simulink model "HLS_design"  (R2023a)
settings: Solver=VariableStepAuto  StartTime=0.0  StopTime=0  RelTol=1e-3  EnableMultiTasking=on
undefined symbols (not defined in the file): A, AXI4, N, Stream, xc7k325tffg900
libraries: hlsBasic x2, Sobeledge_lib x2, dspvision x1, vmcUtilities x1, hlsUtilities x1, visionsinks x1
settings Model: Creator=dvancamp  LastModifiedBy=robg
settings SolverCC: AlgebraicLoopSolver=TrustRegion
settings DataIOCC: LimitDataPoints=on  ReturnWorkspaceOutputs=off
settings OptimizationCC: LifeSpan=inf
settings DebuggingCC: UnconnectedInputMsg=warning  UnconnectedOutputMsg=warning  UnconnectedLineMsg=warning  AllowSymbolicDim=off  SFUnexpectedBacktrackingDiag=warning  SFNoUnconditionalDefaultTransitionDiag=warning  ArithmeticOperatorsInVariantConditions=warning
settings ModelReferenceCC: EnableRefExpFcnMdlSchedulingChecks=on  PropagateSignalLabelsOutOfModel=off
settings SFSimCC: SimUseLocalCustomCode=off  CustomCodeUndefinedFunction=UseInterfaceOnly
settings RTWCC: RTWUseLocalCustomCode=off
settings CodeAppCC: StateflowObjectComments=on
settings GRTTargetCC: TargetLangStandard=C89/C90 (ANSI)
settings ConfigComp: CovMetricSettings=dw  CovSaveCumulativeToWorkspaceVar=on  CovSaveSingleToWorkspaceVar=on  CovExternalEMLEnable=off

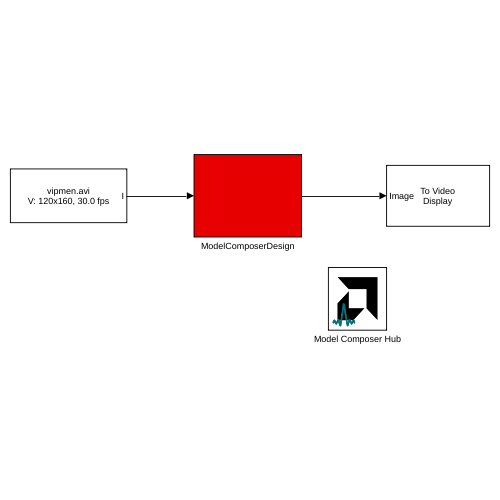
[thumbnail: Simulink's stored preview of the top-level diagram]
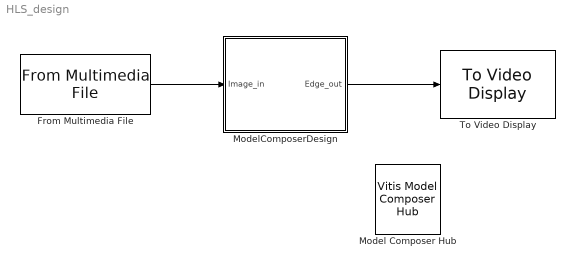
== system HLS_design ==
  From Multimedia File : dspvision/From Multimedia File  inputFilename=vipmen.avi  readRange=[1 Inf]  loop=on  numPlays=inf  outputStreams=Video only  videoDataType=uint8  audioDataType=double  inheritSampleTime=off  userDefinedSampleTime=1/30  noAudioOutput=off  isIntensityVideo=off  fourcc=Intensity  colorVideoFormat=One multidimensional signal  outputEOF=off  dataOrg=Column-major  audioFrameSize=1024  computeAudioFrameSize=off  outSamplingMode=Sample based
  Model Composer Hub : vmcUtilities/Vitis Model Composer Hub  Tag=genX  Description=Performs multiplication  CodeGeneration=off  SubsystemName=ModelComposerDesign  StartColumn=1  NumberOfColumns=1  TargetDirectory=code_HLS  exportDesign=off  analyzeDesign=off  validateDesignOnHw=off  ExportType=System Generator  IpVendor=xilinx.com  IpLibrary=hls  IpVersion=1.0  IpHWLanguage=Verilog  AieCompilerOptions={}  AieSimulatorOptions={}  CreateTestbench=off  TestbenchStackSize=10  RunRtlSim=off  RunCSim=off  RunAieSim=off  AieSimTimeout=50000  RunAieSimProfiling=off  LaunchVitisAnalyzer=off  PlotOutput=off  RunX86Sim=on  X86SimTimeout=10  GenHwImage=off  GenLibadfXo=off  GenHwValidationCode=off  PlatformType=Not Specified  HwSystemType=Baremetal  HwValidationTarget=hw  ProjDevice=Kintex-7 KC705 Evaluation Platform (xc7k325tffg900-2)  ProjDevicePart=xc7k325tffg900-2  SamplePeriod=1  ClockFrequency=200  DataPathParallelism=1  xilinxfamily=Kintex7  part=xc7k325t  speed=-3  package=fbg676  directory=./netlist  testbench=off  incr_netlist=off  synthesis_tool=Vivado  clock_wrapper=Clock Enables  dbl_ovrd=According to Block Masks  dcm_input_clock_period=10  sysclk_period=10  simulink_period=1  eval_field=0  LogFileName=''  NThreads=4
  ModelComposerDesign : Subsystem
  To Video Display : visionsinks/To Video Display  windowSizeMode=True size (1:1)  openAtMdlStart=on  fullScreen=off  videoWindowX=1256  videoWindowY=514  saveWindowSize=off  videoWindowWidth=160  videoWindowHeight=120  inputColorFormat=RGB  inputType=Obsolete  imagePorts=One multidimensional signal  OutputDevice=On-screen video monitor  dataOrg=Column-major  isWindowOpen=off
  wires:
  From Multimedia File/1 -> ModelComposerDesign/1(Image_in)
  ModelComposerDesign/1(Edge_out) -> To Video Display/1

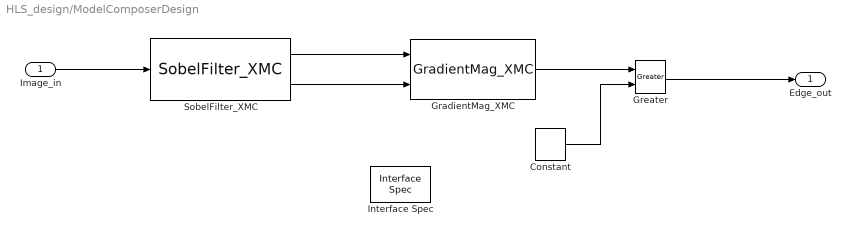
== system HLS_design/ModelComposerDesign ==
  Image_in : Inport
  Constant : hlsBasic/Constant  Description=Performs multiplication  Value=130  VectorParams1D=off  SampleTime=-1  OutDataType=int16  TypeExp=''  Signedness=Signed  WordLength=16  FractionalLength=10  RoundingMode=Truncation to minus infinity  OverflowMode=Wrap around
  GradientMag_XMC : Sobeledge_lib/GradientMag_XMC  LibraryFunction=GradientMag_XMC  IncludeFiles={'GradientMag_Wrap.h'}  SourceFiles={}  IncludeDirectories={'./include'}  TemplateParams={'int ROWS'; 'int COLS'; 'int NPC'}  FunctionParamTypes={xmcDataType('void'); xmcDataType('uint16_t'); xmcDataType('uint16_t'); xmcDataType('uint16_t'); xmcDataType('int')}  FunctionParamPassbys={0.000000000000000000e+00; 0.000000000000000000e+00; 0.000000000000000000e+00; 0.000000000000000000e+00; 0.000000000000000000e+00}  FunctionParamDimensions={'1'; '[ROWS][COLS]'; '[ROWS][COLS]'; '[ROWS][COLS]'; '1'}  FunctionParamNames={'return'; 'inX'; 'inY'; 'Out'; 'NPC'}  FunctionParamDir={0.000000000000000000e+00; 1.000000000000000000e+00; 1.000000000000000000e+00; 2.000000000000000000e+00; 3.000000000000000000e+00}  FunctionParamSupportsStreaming={true; true; true; true; true}  BufferDepth={'0'}  FunctionParamValues={'0'; '0'; '0'; '0'; '0'}  ThroughputFactors={''}  NPC=1
  Greater : hlsBasic/Greater  Description=Performs multiplication
  Interface Spec : hlsUtilities/Interface Spec  Return=No block-level I/O protocol@@  InportInterfaces={'AXI4-Stream@@@N/A@N/A'}  InportHandles={3.610633544921875000e+02}  InportNames={'Image_in'}  OutportInterfaces={'AXI4-Stream@@@N/A@N/A'}  OutportHandles={3.780644531250000000e+02}  OutportNames={'Edge_out'}  Mode=No block-level I/O protocol  InName1=Image_in  InMode1=AXI4-Stream  InVFormat1=N/A  InVComponent1=N/A  InMode2=Default  InVFormat2=N/A  InVComponent2=N/A  InMode3=Default  InVFormat3=N/A  InVComponent3=N/A  InMode4=Default  InVFormat4=N/A  InVComponent4=N/A  InMode5=Default  InVFormat5=N/A  InVComponent5=N/A  InMode6=Default  InVFormat6=N/A  InVComponent6=N/A  InMode7=Default  InVFormat7=N/A  InVComponent7=N/A  InMode8=Default  InVFormat8=N/A  InVComponent8=N/A  OutName1=Edge_out  OutMode1=AXI4-Stream  OutVFormat1=N/A  OutVComponent1=N/A  OutMode2=Default  OutVFormat2=N/A  OutVComponent2=N/A  OutMode3=Default  OutVFormat3=N/A  OutVComponent3=N/A  OutMode4=Default  OutVFormat4=N/A  OutVComponent4=N/A  OutMode5=Default  OutVFormat5=N/A  OutVComponent5=N/A  OutMode6=Default  OutVFormat6=N/A  OutVComponent6=N/A  OutMode7=Default  OutVFormat7=N/A  OutVComponent7=N/A  OutMode8=Default  OutVFormat8=N/A  OutVComponent8=N/A
  SobelFilter_XMC : Sobeledge_lib/SobelFilter_XMC  LibraryFunction=SobelFilter_XMC  IncludeFiles={'sobelfilter_Wrap.h'}  SourceFiles={}  IncludeDirectories={'./include'}  TemplateParams={'int ROWS'; 'int COLS'; 'int NPC'}  FunctionParamTypes={xmcDataType('void'); xmcDataType('uint8_t'); xmcDataType('uint16_t'); xmcDataType('uint16_t'); xmcDataType('int')}  FunctionParamPassbys={0.000000000000000000e+00; 0.000000000000000000e+00; 0.000000000000000000e+00; 0.000000000000000000e+00; 0.000000000000000000e+00}  FunctionParamDimensions={'1'; '[ROWS][COLS]'; '[ROWS][COLS]'; '[ROWS][COLS]'; '1'}  FunctionParamNames={'return'; 'in'; 'outX'; 'outY'; 'NPC'}  FunctionParamDir={0.000000000000000000e+00; 1.000000000000000000e+00; 2.000000000000000000e+00; 2.000000000000000000e+00; 3.000000000000000000e+00}  FunctionParamSupportsStreaming={true; true; true; true; true}  BufferDepth={'0'}  FunctionParamValues={'0'; '0'; '0'; '0'; '0'}  ThroughputFactors={''}  NPC=1
  Edge_out : Outport
  wires:
  Greater/1 -> Edge_out/1
  Image_in/1 -> SobelFilter_XMC/1
  SobelFilter_XMC/1 -> GradientMag_XMC/1
  SobelFilter_XMC/2 -> GradientMag_XMC/2
  GradientMag_XMC/1 -> Greater/1
  Constant/1 -> Greater/2
